simulink model "mass_spring_damper_model"  (R2017b)
settings: Solver=VariableStepAuto  StartTime=2.0  StopTime=20.0  RelTol=1e-3
values from neighbouring files (symbols this model uses):
  b = randi([1,1e1])    [EGH445_Computer_Lab_1.m]    (also in mass_spring_damper_script.m = 1; sim_msd_diff_solvers.m = 100)
  k = 1    [mass_spring_damper_script.m]
  m = 0.15    [CP_ContrSys_Lin_a_Mainfile_n9329013.m]    (also in CP_ContrSys_Lin_b_Mainfile_n9329013.m; MainFile_9329013.m; MainFile_Linearised_a_9329013.m; MainFile_Linearised_b_9329013.m)
  stepf = 0    [mass_spring_damper_script.m]    (also in mymodel_sim.m = 10)
  stepi = 2    [mass_spring_damper_script.m]    (also in mymodel_sim.m = 0)
  stept = 1    [mass_spring_damper_script.m]    (also in mymodel_sim.m)
  z1_0 = 0.8    [mass_spring_damper_script.m]
  z2_0 = 0.7    [mass_spring_damper_script.m]
settings Model: Creator=Koh Kim Hai  LastModifiedBy=Koh Kim Hai

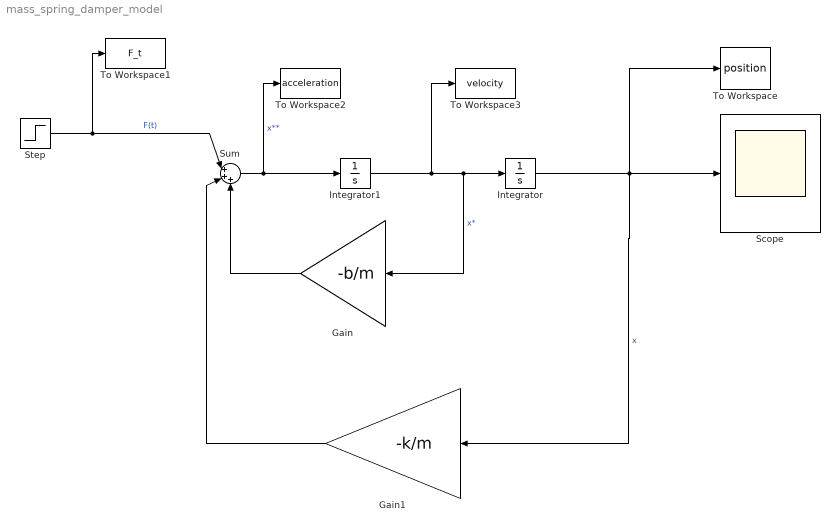
== system mass_spring_damper_model ==
  Gain : Gain  Gain=-b/m
  Gain1 : Gain  Gain=-k/m
  Integrator : Integrator  InitialCondition=z2_0
  Integrator1 : Integrator  InitialCondition=z1_0
  Scope : Scope
  Step : Step  Time=stept  Before=stepi  After=stepf  SampleTime=0
  Sum : Sum  Inputs=|+++
  To Workspace : ToWorkspace  VariableName=position  SampleTime=-1
      settings: Save2DSignal=2-D array (concatenate along first dimension)
  To Workspace1 : ToWorkspace  VariableName=F_t  SampleTime=-1
  To Workspace2 : ToWorkspace  VariableName=acceleration  SampleTime=-1
  To Workspace3 : ToWorkspace  VariableName=velocity  SampleTime=-1
  wires:
  Step/1 -> To Workspace1/1, Sum/1  "F(t)"
  Sum/1 -> To Workspace2/1, Integrator1/1  "x**"
  Gain1/1 -> Sum/2
  Gain/1 -> Sum/3
  Integrator1/1 -> To Workspace3/1, Gain/1, Integrator/1  "x*"
  Integrator/1 -> Gain1/1, Scope/1, To Workspace/1  "x"
